simulink model "Thermal_Model"  (Simulink 8.8)
settings: Solver=ode4  StartTime=0  StopTime=3600  FixedStep=1e-1  RelTol=1e-3  EnableMultiTasking=on
undefined symbols (not defined in the file or in its folder): sigbuilder_block
settings Model: Creator=torres  LastModifiedBy=jarvela7
settings DataIOCC: LimitDataPoints=off  SaveTime=off
settings OptimizationCC: ExpressionDepthLimit=2147483647
settings DebuggingCC: SolverPrmCheckMsg=warning
settings GRTTargetCC: CombineOutputUpdateFcns=on  GRTInterface=off
settings ConfigComp: CovSFcnEnable=off

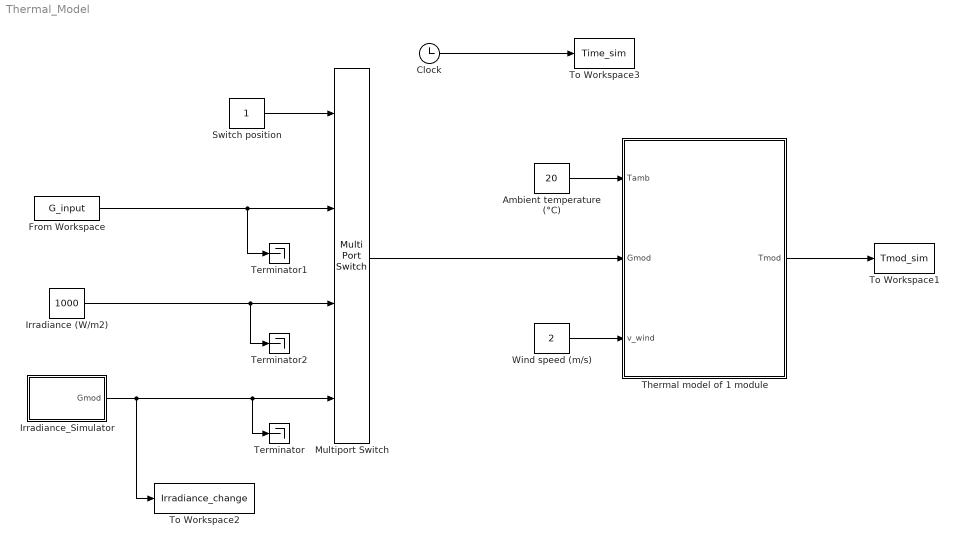
== system Thermal_Model ==
  Ambient temperature (°C) : Constant  Value=20
  Clock : Clock
  From Workspace : FromWorkspace  VariableName=G_input  SampleTime=0
  Irradiance (W/m2) : Constant  Value=1000
  Irradiance_Simulator : Subsystem  Tag=STV Subsys  LoadFcn=sigbuilder_block('load');  StartFcn=sigbuilder_block('start');  StopFcn=sigbuilder_block('stop');  ClipboardFcn=sigbuilder_block('clipboard');  mask(Sigbuilder block){tuvar=[0:10]}
      mask help: Simulink:masks:SigbuilderBlock_MD
      mask init:
      | if ~strcmp(get_param(bdroot(gcbh),'SimulationStatus'),'stopped') tuvar = sigbuilder_block('maskInit'); end
      settings: CopyFcn=sigbuilder_block('copy');  DeleteFcn=sigbuilder_block('delete');  ModelCloseFcn=sigbuilder_block('modelClose');  PreSaveFcn=sigbuilder_block('preSave');  PauseFcn=sigbuilder_block('pause');  ContinueFcn=sigbuilder_block('continue');  NameChangeFcn=sigbuilder_block('namechange');  OpenFcn=sigbuilder_block('open',[6 36 1068 576 ]);  CloseFcn=sigbuilder_block('close');
      mask Display: plot(0, 0, 100, 100,[2, 2, 32, 32, 2], [68, 8, 8, 68, 68],[32, 2], [38, 38], [32, 19, 2],[53, 60, 44], [32, 17, 17, 2],[16, 16, 31, 31]);txt = getActiveGroup(gcbh);text(2, 100, txt,'verticalAlignment', 'top');
  Multiport Switch : MultiPortSwitch
  Switch position : Constant
  Terminator : Terminator
  Terminator1 : Terminator
  Terminator2 : Terminator
  Thermal model of 1 module : Subsystem  mask{Tini=25, Cmod=20700}
      mask prompts: Tini "Initial module temperature (Celsius)"; Cmod "Heat capacitance (J/K)"
  To Workspace1 : ToWorkspace  VariableName=Tmod_sim  SampleTime=-1
  To Workspace2 : ToWorkspace  VariableName=Irradiance_change  SampleTime=-1
  To Workspace3 : ToWorkspace  VariableName=Time_sim  SampleTime=-1
  Wind speed (m/s) : Constant  Value=2
  wires:
  Thermal model of 1 module/1(Tmod) -> To Workspace1/1
  Clock/1 -> To Workspace3/1
  Ambient temperature (°C)/1 -> Thermal model of 1 module/1(Tamb)
  Wind speed (m/s)/1 -> Thermal model of 1 module/3(v_wind)
  From Workspace/1 -> Terminator1/1, Multiport Switch/2
  Irradiance (W/m2)/1 -> Multiport Switch/3, Terminator2/1
  Irradiance_Simulator/1(Gmod) -> To Workspace2/1, Terminator/1, Multiport Switch/4
  Multiport Switch/1 -> Thermal model of 1 module/2(Gmod)
  Switch position/1 -> Multiport Switch/1

== system Thermal_Model/Irradiance_Simulator ==
  Demux : Demux  Tag=STV Demux  Outputs=1
  FromWs : FromWorkspace  Tag=STV FromWs  VariableName=tuvar  SampleTime=0  SigBuilderData=DataTag0  VnvData=DataTag1
      SigBuilderData=|
      | common.afterFinalStr = 'Extrapolate'
      | common.sampleTime = 0
      | dataSet.timeRange = [0 1800]
      | dataSet.name = 'Group 1'
      | sbobj.Groups.Name = 'Group 1'
      | sbobj.Groups.Signals.Name = 'Gmod'
      | sbobj.Groups.Signals.XData = [0 400 400 1800]
      | sbobj.Groups.Signals.YData = [200 200 1000 1000]
      | sbobj.Groups.TimeRange = [0 1800]
  Gmod : Outport  Tag=STV Outport
  wires:
  Demux/1 -> Gmod/1
  FromWs/1 -> Demux/1

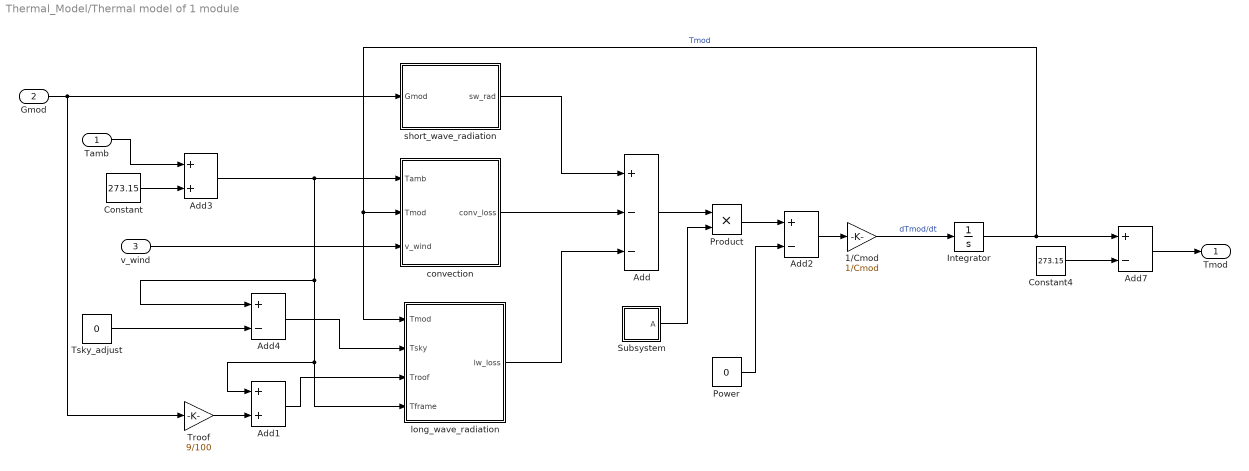
== system Thermal_Model/Thermal model of 1 module ==
  Tamb : Inport
  Gmod : Inport  Port=2
  v_wind : Inport  Port=3
  1/Cmod : Gain  Gain=1/Cmod
  Add : Sum  Inputs=+--
  Add1 : Sum
  Add2 : Sum  Inputs=+-
  Add3 : Sum
  Add4 : Sum  Inputs=+-
  Add7 : Sum  Inputs=+-
  Constant : Constant  Value=273.15
  Constant4 : Constant  Value=273.15
  Integrator : Integrator  InitialCondition=Tini+273  LimitOutput=on  UpperSaturationLimit=373  LowerSaturationLimit=173
  Power : Constant  Value=0
  Product : Product  RndMeth=Zero
  Subsystem : Subsystem
  Troof : Gain  Gain=9/100
  Tsky_adjust : Constant  Value=0
  convection : Subsystem
  long_wave_radiation : Subsystem
  short_wave_radiation : Subsystem
  Tmod : Outport
  wires:
  v_wind/1 -> convection/3(v_wind)
  Gmod/1 -> short_wave_radiation/1(Gmod), Troof/1
  short_wave_radiation/1(sw_rad) -> Add/1
  convection/1(conv_loss) -> Add/2
  long_wave_radiation/1(lw_loss) -> Add/3
  Add/1 -> Product/1
  Subsystem/1(A) -> Product/2
  Add2/1 -> 1/Cmod/1
  Product/1 -> Add2/1
  Add3/1 -> convection/1(Tamb), Add4/1, long_wave_radiation/4(Tframe), Add1/1
  Tamb/1 -> Add3/1
  Constant/1 -> Add3/2
  Tsky_adjust/1 -> Add4/2
  Add4/1 -> long_wave_radiation/2(Tsky)
  Add1/1 -> long_wave_radiation/3(Troof)
  Constant4/1 -> Add7/2
  Add7/1 -> Tmod/1
  1/Cmod/1 -> Integrator/1  "dTmod/dt"
  Integrator/1 -> Add7/1, convection/2(Tmod), long_wave_radiation/1(Tmod)  "Tmod"
  Troof/1 -> Add1/2
  Power/1 -> Add2/2

== system Thermal_Model/Thermal model of 1 module/Subsystem ==
  H : Constant  Value=0.156*6
  Product : Product  RndMeth=Zero
  W : Constant  Value=0.156*9
  A : Outport
  wires:
  Product/1 -> A/1
  W/1 -> Product/2
  H/1 -> Product/1

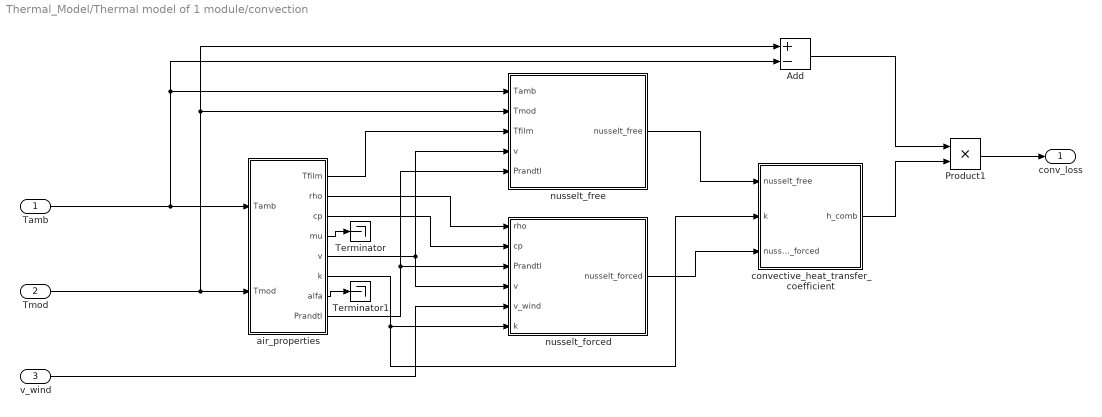
== system Thermal_Model/Thermal model of 1 module/convection ==
  Tamb : Inport
  Tmod : Inport  Port=2  OutMin=225
  v_wind : Inport  Port=3
  Add : Sum  Inputs=+-
  Product1 : Product  RndMeth=Zero
  Terminator : Terminator
  Terminator1 : Terminator
  air_properties : Subsystem
  convective_heat_transfer_coefficient : Subsystem
  nusselt_forced : Subsystem
  nusselt_free : Subsystem
  conv_loss : Outport
  wires:
  air_properties/7(alfa) -> Terminator1/1
  air_properties/4(mu) -> Terminator/1
  nusselt_forced/1(nusselt_forced) -> convective_heat_transfer_coefficient/3(nusselt_forced)
  nusselt_free/1(nusselt_free) -> convective_heat_transfer_coefficient/1(nusselt_free)
  air_properties/6(k) -> nusselt_forced/6(k), convective_heat_transfer_coefficient/2(k)
  v_wind/1 -> nusselt_forced/5(v_wind)
  air_properties/3(cp) -> nusselt_forced/2(cp)
  air_properties/2(rho) -> nusselt_forced/1(rho)
  air_properties/8(Prandtl) -> nusselt_forced/3(Prandtl), nusselt_free/5(Prandtl)
  air_properties/5(v) -> nusselt_free/4(v), nusselt_forced/4(v)
  air_properties/1(Tfilm) -> nusselt_free/3(Tfilm)
  Tmod/1 -> air_properties/2(Tmod), nusselt_free/2(Tmod), Add/1
  Tamb/1 -> air_properties/1(Tamb), nusselt_free/1(Tamb), Add/2
  Add/1 -> Product1/1
  convective_heat_transfer_coefficient/1(h_comb) -> Product1/2
  Product1/1 -> conv_loss/1

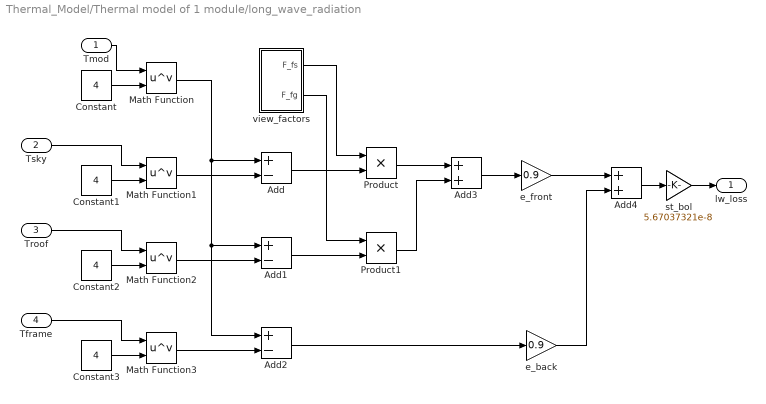
== system Thermal_Model/Thermal model of 1 module/long_wave_radiation ==
  Tmod : Inport
  Tsky : Inport  Port=2
  Troof : Inport  Port=3
  Tframe : Inport  Port=4
  Add : Sum  Inputs=+-
  Add1 : Sum  Inputs=+-
  Add2 : Sum  Inputs=+-
  Add3 : Sum
  Add4 : Sum
  Constant{,1..3} (4 alike) : Constant  Value=4
  Math Function{,1..3} (4 alike) : Math  Operator=pow  SaturateOnIntegerOverflow=on
  Product : Product  RndMeth=Zero
  Product1 : Product  RndMeth=Zero
  e_back : Gain  Gain=0.9
  e_front : Gain  Gain=0.9
  st_bol : Gain  Gain=5.67037321e-8
  view_factors : Subsystem
  lw_loss : Outport
  wires:
  e_back/1 -> Add4/2
  e_front/1 -> Add4/1
  Add2/1 -> e_back/1
  Add3/1 -> e_front/1
  Product1/1 -> Add3/2
  Product/1 -> Add3/1
  Add1/1 -> Product1/2
  view_factors/2(F_fg) -> Product1/1
  Add/1 -> Product/2
  view_factors/1(F_fs) -> Product/1
  Math Function3/1 -> Add2/2
  Math Function2/1 -> Add1/2
  Math Function1/1 -> Add/2
  Math Function/1 -> Add/1, Add1/1, Add2/1
  Tframe/1 -> Math Function3/1
  Constant3/1 -> Math Function3/2
  Troof/1 -> Math Function2/1
  Constant2/1 -> Math Function2/2
  Tsky/1 -> Math Function1/1
  Constant1/1 -> Math Function1/2
  Constant/1 -> Math Function/2
  Add4/1 -> st_bol/1
  Tmod/1 -> Math Function/1
  st_bol/1 -> lw_loss/1

== system Thermal_Model/Thermal model of 1 module/short_wave_radiation ==
  Gmod : Inport
  absorptivity : Gain  Gain=0.9
  sw_rad : Outport
  wires:
  Gmod/1 -> absorptivity/1
  absorptivity/1 -> sw_rad/1

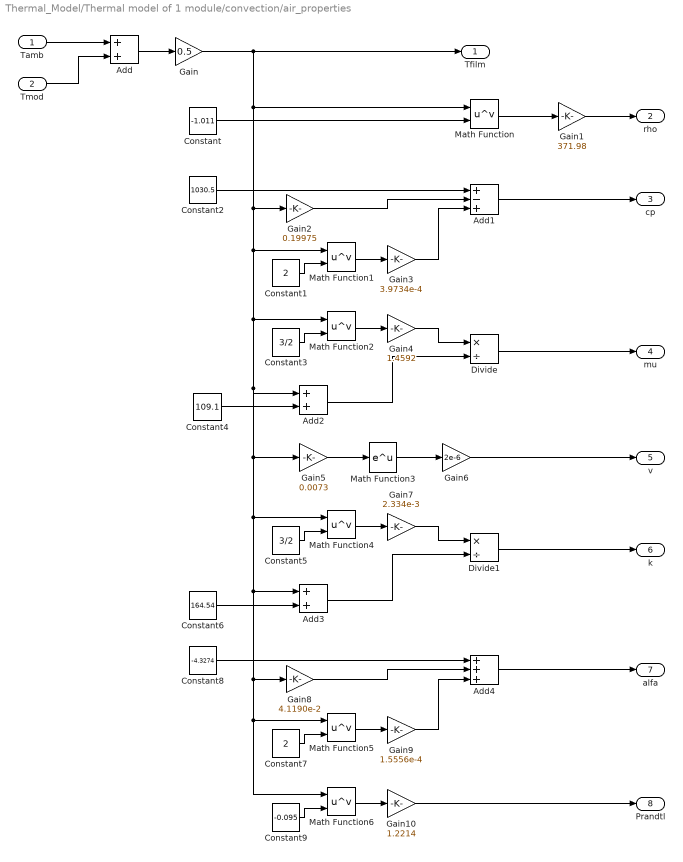
== system Thermal_Model/Thermal model of 1 module/convection/air_properties ==
  Tamb : Inport
  Tmod : Inport  Port=2
  Add : Sum
  Add1 : Sum  Inputs=+-+
  Add2 : Sum
  Add3 : Sum
  Add4 : Sum  Inputs=+++
  Constant : Constant  Value=-1.011
  Constant1 : Constant  Value=2
  Constant2 : Constant  Value=1030.5
  Constant3 : Constant  Value=3/2
  Constant4 : Constant  Value=109.1
  Constant5 : Constant  Value=3/2
  Constant6 : Constant  Value=164.54
  Constant7 : Constant  Value=2
  Constant8 : Constant  Value=-4.3274
  Constant9 : Constant  Value=-0.095
  Divide : Product  Inputs=*/
  Divide1 : Product  Inputs=*/
  Gain : Gain  Gain=0.5
  Gain1 : Gain  Gain=371.98
  Gain10 : Gain  Gain=1.2214
  Gain2 : Gain  Gain=0.19975
  Gain3 : Gain  Gain=3.9734e-4
  Gain4 : Gain  Gain=1.4592
  Gain5 : Gain  Gain=0.0073
  Gain6 : Gain  Gain=2e-6
  Gain7 : Gain  Gain=2.334e-3
  Gain8 : Gain  Gain=4.1190e-2
  Gain9 : Gain  Gain=1.5556e-4
  Math Function{,1..2,4..6} (6 alike) : Math  Operator=pow  SaturateOnIntegerOverflow=on
  Math Function3 : Math  SaturateOnIntegerOverflow=on
  Tfilm : Outport
  rho : Outport  Port=2
  cp : Outport  Port=3
  mu : Outport  Port=4
  v : Outport  Port=5
  k : Outport  Port=6
  alfa : Outport  Port=7
  Prandtl : Outport  Port=8
  wires:
  Tamb/1 -> Add/1
  Tmod/1 -> Add/2
  Add/1 -> Gain/1
  Gain/1 -> Math Function/1, Gain2/1, Math Function1/1, Math Function2/1, Add2/1, Gain5/1, Math Function4/1, Add3/1, Gain8/1, Math Function5/1, Math Function6/1, Tfilm/1
  Constant/1 -> Math Function/2
  Math Function/1 -> Gain1/1
  Gain1/1 -> rho/1
  Constant1/1 -> Math Function1/2
  Constant2/1 -> Add1/1
  Gain2/1 -> Add1/2
  Math Function1/1 -> Gain3/1
  Gain3/1 -> Add1/3
  Add1/1 -> cp/1
  Constant3/1 -> Math Function2/2
  Math Function2/1 -> Gain4/1
  Constant4/1 -> Add2/2
  Gain4/1 -> Divide/1
  Add2/1 -> Divide/2
  Divide/1 -> mu/1
  Gain5/1 -> Math Function3/1
  Math Function3/1 -> Gain6/1
  Gain6/1 -> v/1
  Constant5/1 -> Math Function4/2
  Math Function4/1 -> Gain7/1
  Constant7/1 -> Math Function5/2
  Constant8/1 -> Add4/1
  Gain8/1 -> Add4/2
  Math Function5/1 -> Gain9/1
  Gain9/1 -> Add4/3
  Add4/1 -> alfa/1
  Constant9/1 -> Math Function6/2
  Math Function6/1 -> Gain10/1
  Gain10/1 -> Prandtl/1
  Constant6/1 -> Add3/2
  Add3/1 -> Divide1/2
  Gain7/1 -> Divide1/1
  Divide1/1 -> k/1

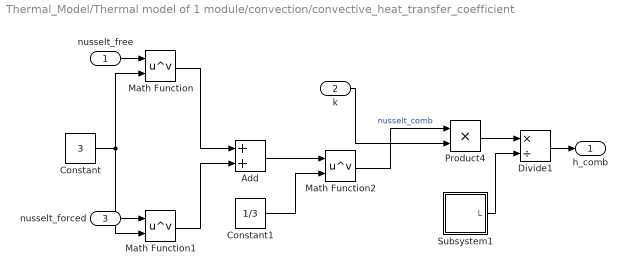
== system Thermal_Model/Thermal model of 1 module/convection/convective_heat_transfer_coefficient ==
  nusselt_free : Inport
  k : Inport  Port=2
  nusselt_forced : Inport  Port=3
  Add : Sum
  Constant : Constant  Value=3
  Constant1 : Constant  Value=1/3
  Divide1 : Product  Inputs=*/
  Math Function : Math  Operator=pow  SaturateOnIntegerOverflow=on
  Math Function1 : Math  Operator=pow  SaturateOnIntegerOverflow=on
  Math Function2 : Math  Operator=pow  SaturateOnIntegerOverflow=on
  Product4 : Product  RndMeth=Zero
  Subsystem1 : Subsystem
  h_comb : Outport
  wires:
  Constant/1 -> Math Function/2, Math Function1/2
  Math Function/1 -> Add/1
  Math Function1/1 -> Add/2
  Add/1 -> Math Function2/1
  Constant1/1 -> Math Function2/2
  Product4/1 -> Divide1/1
  Math Function2/1 -> Product4/1  "nusselt_comb"
  Subsystem1/1(L) -> Divide1/2
  k/1 -> Product4/2
  nusselt_free/1 -> Math Function/1
  Divide1/1 -> h_comb/1
  nusselt_forced/1 -> Math Function1/1

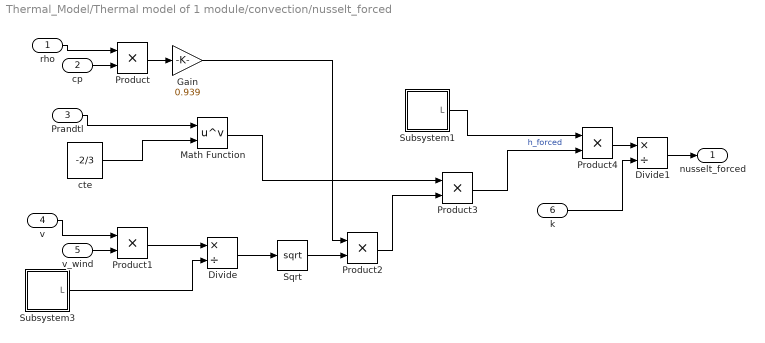
== system Thermal_Model/Thermal model of 1 module/convection/nusselt_forced ==
  rho : Inport
  cp : Inport  Port=2
  Prandtl : Inport  Port=3
  v : Inport  Port=4
  v_wind : Inport  Port=5
  k : Inport  Port=6
  Divide : Product  Inputs=*/
  Divide1 : Product  Inputs=*/
  Gain : Gain  Gain=0.939
  Math Function : Math  Operator=pow  SaturateOnIntegerOverflow=on
  Product{,1..4} (5 alike) : Product  RndMeth=Zero
  Sqrt : Sqrt  SaturateOnIntegerOverflow=on
  Subsystem1 : Subsystem
  Subsystem3 : Subsystem
  cte : Constant  Value=-2/3
  nusselt_forced : Outport
  wires:
  Product/1 -> Gain/1
  Product1/1 -> Divide/1
  Subsystem3/1(L) -> Divide/2
  Divide/1 -> Sqrt/1
  Gain/1 -> Product2/1
  Sqrt/1 -> Product2/2
  Product2/1 -> Product3/2
  cte/1 -> Math Function/2
  Math Function/1 -> Product3/1
  Prandtl/1 -> Math Function/1
  v/1 -> Product1/1
  rho/1 -> Product/1
  cp/1 -> Product/2
  v_wind/1 -> Product1/2
  Product3/1 -> Product4/2  "h_forced"
  Subsystem1/1(L) -> Product4/1
  Product4/1 -> Divide1/1
  k/1 -> Divide1/2
  Divide1/1 -> nusselt_forced/1

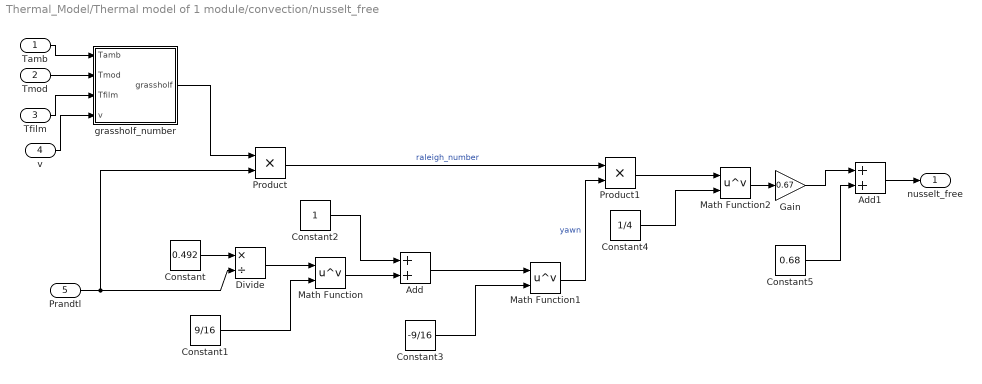
== system Thermal_Model/Thermal model of 1 module/convection/nusselt_free ==
  Tamb : Inport
  Tmod : Inport  Port=2
  Tfilm : Inport  Port=3
  v : Inport  Port=4
  Prandtl : Inport  Port=5
  Add : Sum
  Add1 : Sum
  Constant : Constant  Value=0.492
  Constant1 : Constant  Value=9/16
  Constant2 : Constant
  Constant3 : Constant  Value=-9/16
  Constant4 : Constant  Value=1/4
  Constant5 : Constant  Value=0.68
  Divide : Product  Inputs=*/
  Gain : Gain  Gain=0.67
  Math Function : Math  Operator=pow  SaturateOnIntegerOverflow=on
  Math Function1 : Math  Operator=pow  SaturateOnIntegerOverflow=on
  Math Function2 : Math  Operator=pow  SaturateOnIntegerOverflow=on
  Product : Product  RndMeth=Zero
  Product1 : Product  RndMeth=Zero
  grassholf_number : Subsystem
  nusselt_free : Outport
  wires:
  grassholf_number/1(grassholf) -> Product/1
  Prandtl/1 -> Divide/2, Product/2
  Product/1 -> Product1/1  "raleigh_number"
  Constant/1 -> Divide/1
  Divide/1 -> Math Function/1
  Constant1/1 -> Math Function/2
  Math Function/1 -> Add/2
  Constant2/1 -> Add/1
  Add/1 -> Math Function1/1
  Constant3/1 -> Math Function1/2
  Math Function1/1 -> Product1/2  "yawn"
  Product1/1 -> Math Function2/1
  Constant4/1 -> Math Function2/2
  Math Function2/1 -> Gain/1
  Gain/1 -> Add1/1
  Constant5/1 -> Add1/2
  Add1/1 -> nusselt_free/1
  Tamb/1 -> grassholf_number/1(Tamb)
  Tmod/1 -> grassholf_number/2(Tmod)
  Tfilm/1 -> grassholf_number/3(Tfilm)
  v/1 -> grassholf_number/4(v)

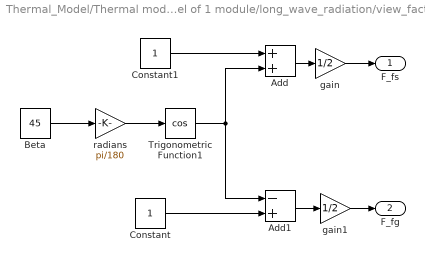
== system Thermal_Model/Thermal model of 1 module/long_wave_radiation/view_factors ==
  Add : Sum
  Add1 : Sum  Inputs=-+
  Beta : Constant  Value=45
  Constant : Constant
  Constant1 : Constant
  Trigonometric Function1 : Trigonometry  Operator=cos
  gain : Gain  Gain=1/2
  gain1 : Gain  Gain=1/2
  radians : Gain  Gain=pi/180
  F_fs : Outport
  F_fg : Outport  Port=2
  wires:
  Beta/1 -> radians/1
  radians/1 -> Trigonometric Function1/1
  Trigonometric Function1/1 -> Add/2, Add1/1
  Constant1/1 -> Add/1
  Constant/1 -> Add1/2
  Add/1 -> gain/1
  Add1/1 -> gain1/1
  gain1/1 -> F_fg/1
  gain/1 -> F_fs/1

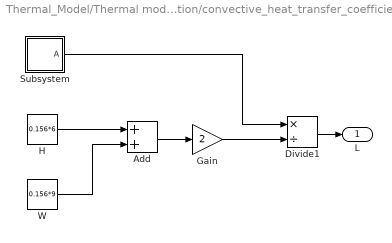
== system Thermal_Model/Thermal model of 1 module/convection/convective_heat_transfer_coefficient/Subsystem1 ==
  Add : Sum
  Divide1 : Product  Inputs=*/
  Gain : Gain  Gain=2
  H : Constant  Value=0.156*6
  Subsystem : Subsystem
  W : Constant  Value=0.156*9
  L : Outport
  wires:
  H/1 -> Add/1
  W/1 -> Add/2
  Add/1 -> Gain/1
  Gain/1 -> Divide1/2
  Subsystem/1(A) -> Divide1/1
  Divide1/1 -> L/1

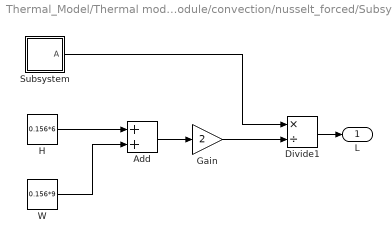
== system Thermal_Model/Thermal model of 1 module/convection/nusselt_forced/Subsystem1 ==
  Add : Sum
  Divide1 : Product  Inputs=*/
  Gain : Gain  Gain=2
  H : Constant  Value=0.156*6
  Subsystem : Subsystem
  W : Constant  Value=0.156*9
  L : Outport
  wires:
  H/1 -> Add/1
  W/1 -> Add/2
  Add/1 -> Gain/1
  Gain/1 -> Divide1/2
  Subsystem/1(A) -> Divide1/1
  Divide1/1 -> L/1

== system Thermal_Model/Thermal model of 1 module/convection/nusselt_forced/Subsystem3 ==
  Add : Sum
  Divide1 : Product  Inputs=*/
  Gain : Gain  Gain=2
  H : Constant  Value=0.156*6
  Subsystem : Subsystem
  W : Constant  Value=0.156*9
  L : Outport
  wires:
  H/1 -> Add/1
  W/1 -> Add/2
  Add/1 -> Gain/1
  Gain/1 -> Divide1/2
  Subsystem/1(A) -> Divide1/1
  Divide1/1 -> L/1

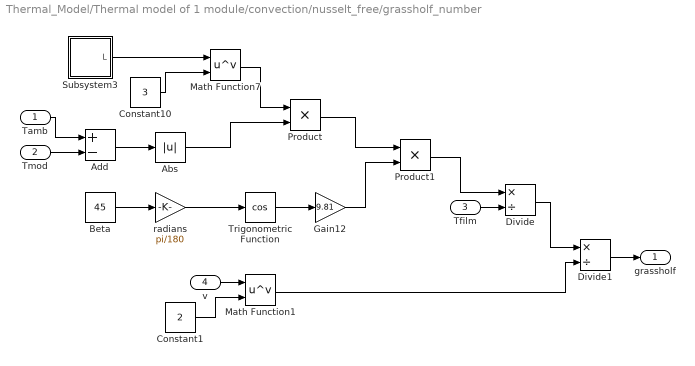
== system Thermal_Model/Thermal model of 1 module/convection/nusselt_free/grassholf_number ==
  Tamb : Inport
  Tmod : Inport  Port=2
  Tfilm : Inport  Port=3
  v : Inport  Port=4
  Abs : Abs
  Add : Sum  Inputs=+-
  Beta : Constant  Value=45
  Constant1 : Constant  Value=2
  Constant10 : Constant  Value=3
  Divide : Product  Inputs=*/
  Divide1 : Product  Inputs=*/
  Gain12 : Gain  Gain=9.81
  Math Function1 : Math  Operator=pow  SaturateOnIntegerOverflow=on
  Math Function7 : Math  Operator=pow  SaturateOnIntegerOverflow=on
  Product : Product  RndMeth=Zero
  Product1 : Product  RndMeth=Zero
  Subsystem3 : Subsystem
  Trigonometric Function : Trigonometry  Operator=cos
  radians : Gain  Gain=pi/180
  grassholf : Outport
  wires:
  Constant10/1 -> Math Function7/2
  Beta/1 -> radians/1
  Trigonometric Function/1 -> Gain12/1
  Subsystem3/1(L) -> Math Function7/1
  Add/1 -> Abs/1
  Math Function7/1 -> Product/1
  Abs/1 -> Product/2
  Product/1 -> Product1/1
  Gain12/1 -> Product1/2
  Product1/1 -> Divide/1
  Constant1/1 -> Math Function1/2
  Divide/1 -> Divide1/1
  Math Function1/1 -> Divide1/2
  Tamb/1 -> Add/1
  Tmod/1 -> Add/2
  Tfilm/1 -> Divide/2
  v/1 -> Math Function1/1
  Divide1/1 -> grassholf/1
  radians/1 -> Trigonometric Function/1

== system Thermal_Model/Thermal model of 1 module/convection/convective_heat_transfer_coefficient/Subsystem1/Subsystem ==
  H : Constant  Value=0.156*6
  Product : Product  RndMeth=Zero
  W : Constant  Value=0.156*9
  A : Outport
  wires:
  Product/1 -> A/1
  W/1 -> Product/2
  H/1 -> Product/1

== system Thermal_Model/Thermal model of 1 module/convection/nusselt_forced/Subsystem1/Subsystem ==
  H : Constant  Value=0.156*6
  Product : Product  RndMeth=Zero
  W : Constant  Value=0.156*9
  A : Outport
  wires:
  Product/1 -> A/1
  W/1 -> Product/2
  H/1 -> Product/1

== system Thermal_Model/Thermal model of 1 module/convection/nusselt_forced/Subsystem3/Subsystem ==
  H : Constant  Value=0.156*6
  Product : Product  RndMeth=Zero
  W : Constant  Value=0.156*9
  A : Outport
  wires:
  Product/1 -> A/1
  W/1 -> Product/2
  H/1 -> Product/1

== system Thermal_Model/Thermal model of 1 module/convection/nusselt_free/grassholf_number/Subsystem3 ==
  Add : Sum
  Divide1 : Product  Inputs=*/
  Gain : Gain  Gain=2
  H : Constant  Value=0.156*6
  Subsystem : Subsystem
  W : Constant  Value=0.156*9
  L : Outport
  wires:
  H/1 -> Add/1
  W/1 -> Add/2
  Add/1 -> Gain/1
  Gain/1 -> Divide1/2
  Subsystem/1(A) -> Divide1/1
  Divide1/1 -> L/1

== system Thermal_Model/Thermal model of 1 module/convection/nusselt_free/grassholf_number/Subsystem3/Subsystem ==
  H : Constant  Value=0.156*6
  Product : Product  RndMeth=Zero
  W : Constant  Value=0.156*9
  A : Outport
  wires:
  Product/1 -> A/1
  W/1 -> Product/2
  H/1 -> Product/1
